simulink model "PROYECTO_IV_SIMULINK_II"  (R2020b)
settings: Solver=VariableStepAuto  StartTime=0.0  StopTime=500  RelTol=1e-3
libraries: simulink x1, pid_lib x1
settings Model: Creator=NITRO  LastModifiedBy=NITRO

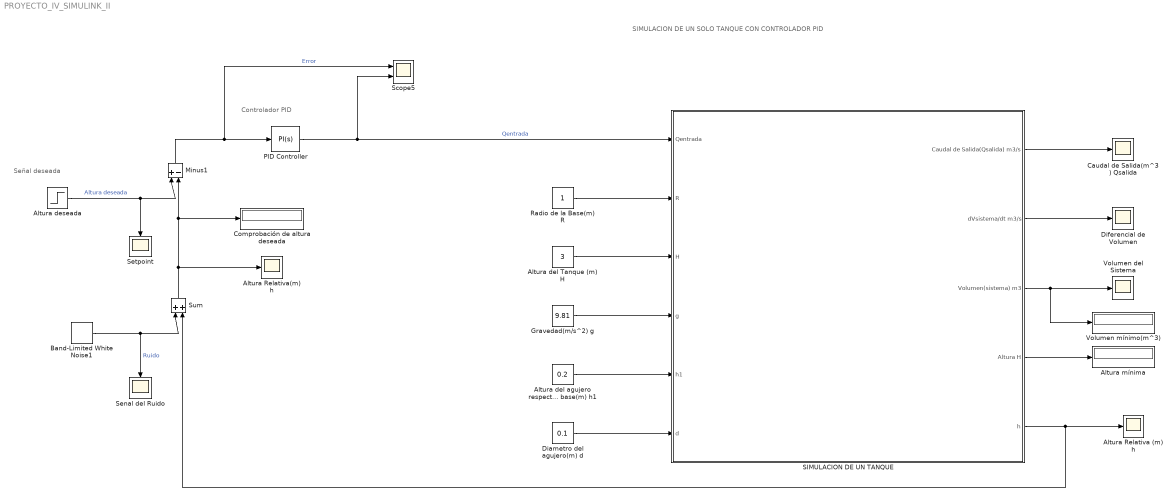
== system PROYECTO_IV_SIMULINK_II ==
  note: SIMULACION DE UN SOLO TANQUE CON CONTROLADOR PID
  note: Señal deseada
  note: Controlador PID
  Altura Relativa (m) h : Scope
  Altura Relativa(m) h : Scope
  Altura del Tanque (m) H : Constant  Value=3
  Altura del agujero respecto de la base(m) h1 : Constant  Value=0.2
  Altura deseada : Step  Time=50  Before=2  After=2.5  SampleTime=0
  Altura mínima : Display
  Band-Limited White Noise1 : simulink/Sources/Band-Limited White Noise  Cov=[0.001]  Ts=0.5  seed=[2525]
  Caudal de Salida(m^3) Qsalida : Scope
  Comprobación de altura deseada : Display
  Diametro del agujero(m) d : Constant  Value=0.1
  Diferencial de Volumen : Scope
  "Gravedad(m/s^2) g " : Constant  Value=9.81
  Minus1 : Sum  Inputs=|+-
  PID Controller : pid_lib/PID Controller  Controller=PI  Form=Parallel  TimeDomain=Continuous-time  UseExternalTs=off  SampleTime=-1  IntegratorMethod=Forward Euler  FilterMethod=Forward Euler  ControllerParametersSource=internal  P=10  I=4  D=0  UseFilter=on  N=0.0363987705373883  TunerSelectOption=Transfer Function Based (PID Tuner App)  InitialConditionSource=internal  InitialConditionForIntegrator=0  InitialConditionForFilter=0  DifferentiatorICPrevScaledInput=0  ExternalReset=none  TrackingMode=off  Kt=1  LimitOutput=on  SatLimitsSource=internal  UpperSaturationLimit=2000  LowerSaturationLimit=0  LinearizeAsGain=on  AntiWindupMode=none  Kb=1  POutMin=[]  POutMax=[]  IOutMin=[]  IOutMax=[]  DOutMin=[]  DOutMax=[]  NOutMin=[]  NOutMax=[]  SumOutMin=[]  SumOutMax=[]  SaturationOutMin=[]  SaturationOutMax=[]  PParamMin=[]  PParamMax=[]  IParamMin=[]  IParamMax=[]  DParamMin=[]  DParamMax=[]  NParamMin=[]  NParamMax=[]  KbParamMin=[]  KbParamMax=[]  KtParamMin=[]  KtParamMax=[]  KbOutMin=[]  KbOutMax=[]  KtOutMin=[]  KtOutMax=[]  IntegratorOutMin=[]  IntegratorOutMax=[]  FilterOutMin=[]  FilterOutMax=[]  SumI1OutMin=[]  SumI1OutMax=[]  SumI2OutMin=[]  SumI2OutMax=[]  SumI3OutMin=[]  SumI3OutMax=[]  SumI4OutMin=[]  SumI4OutMax=[]  SumDOutMin=[]  SumDOutMax=[]  DifferentiatorOutMin=[]  DifferentiatorOutMax=[]  FilterDiffOutCoefMin=[]  FilterDiffOutCoefMax=[]  ReciprocalOutMin=[]  ReciprocalOutMax=[]  SumDenOutMin=[]  SumDenOutMax=[]  SumNumOutMin=[]  SumNumOutMax=[]  DivideOutMin=[]  DivideOutMax=[]  UdiffTsProdOutMin=[]  UdiffTsProdOutMax=[]  NTsProdOutMin=[]  NTsProdOutMax=[]  UintegralTsProdOutMin=[]  UintegralTsProdOutMax=[]  UngainTsProdOutMin=[]  UngainTsProdOutMax=[]  IntegratorContinuousStateAttributes=''  IntegratorStateMustResolveToSignalObject=off  IntegratorRTWStateStorageClass=Auto  FilterContinuousStateAttributes=''  FilterStateMustResolveToSignalObject=off  FilterRTWStateStorageClass=Auto  ParallelPVariant=InternalParameters  IdealPVariant=Disabled  IVariant=InternalParameters  DVariant=Disabled  IntegratorVariant=Continuous  SatVariant=Enabled  AWVariant=Passthrough  PCopyVariant=Disabled  TRVariant=Disabled  FdbkBlocksVariant=Forward  IdealPFdbkVariant=Disabled  SatFdbkVariant=Disabled  DerivativeFilterVariant=Disabled  NVariant=Disabled  NCopyVariant=Disabled_SignalSpec  FilterICVariant=Disabled  IntegratorICVariant=InternalICs  ExternalResetVariant=Disabled  TRSumVariant=Passthrough  SumFdbkVariant=Disabled  SumVariant=Sum_PI  TsampFilterVariant=InternalTs  TsampNgainVariant=Passthrough  TsampIntegralVariant=Passthrough  ExternalSaturationOutDataTypeStr=Inherit: Same as second input
  Radio de la Base(m) R : Constant
  SIMULACION DE UN TANQUE : Subsystem
      mask Display: image('$imagefile'); % Use "Edit Image" on toolstrip to change.
  Scope5 : Scope  NumInputPorts=2
  Senal del Ruido : Scope
  Setpoint : Scope
  Sum : Sum  Inputs=|++
  Volumen del Sistema : Scope
  Volumen mínimo(m^3) : Display
  wires:
  SIMULACION DE UN TANQUE/3(Volumen(sistema) m3) -> Volumen mínimo(m^3)/1, Volumen del Sistema/1
  Radio de la Base(m) R/1 -> SIMULACION DE UN TANQUE/2(R)
  Altura del Tanque (m) H/1 -> SIMULACION DE UN TANQUE/3(H)
  "Gravedad(m/s^2) g "/1 -> SIMULACION DE UN TANQUE/4(g)
  Altura del agujero respecto de la base(m) h1/1 -> SIMULACION DE UN TANQUE/5(h1)
  Diametro del agujero(m) d/1 -> SIMULACION DE UN TANQUE/6(d)
  SIMULACION DE UN TANQUE/2(dVsistema/dt m3/s) -> Diferencial de Volumen/1
  SIMULACION DE UN TANQUE/1(Caudal de Salida(Qsalida) m3/s) -> Caudal de Salida(m^3) Qsalida/1
  SIMULACION DE UN TANQUE/5(h) -> Altura Relativa (m) h/1, Sum/2
  Minus1/1 -> Scope5/1, PID Controller/1  "Error"
  SIMULACION DE UN TANQUE/4(Altura H) -> Altura mínima/1
  Band-Limited White Noise1/1 -> Sum/1, Senal del Ruido/1  "Ruido"
  Altura deseada/1 -> Minus1/1, Setpoint/1  "Altura deseada"
  PID Controller/1 -> SIMULACION DE UN TANQUE/1(Qentrada), Scope5/2  "Qentrada"
  Sum/1 -> Minus1/2, Comprobación de altura deseada/1, Altura Relativa(m) h/1

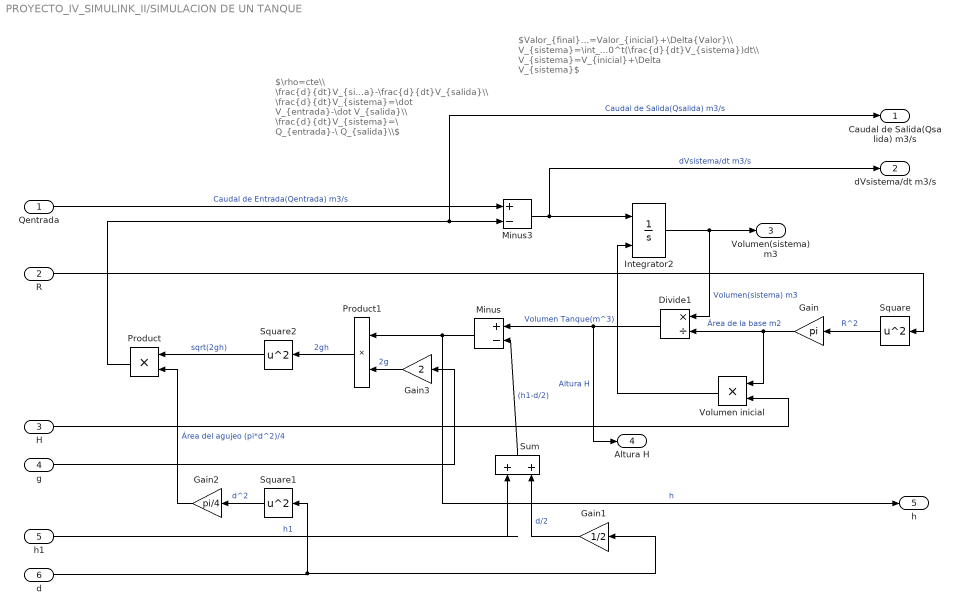
== system PROYECTO_IV_SIMULINK_II/SIMULACION DE UN TANQUE ==
  note: $\rho=cte\\ \frac{d}{dt}V_{sistema}=\frac{d}{dt}V_{entrada}-\frac{d}{dt}V_{salida}\\ \frac{d}{dt}V_{sistema}=\dot V_{entrada}-\dot V_{salida}\\ \frac{d}{dt}V_{sistema}=\ Q_{entrada}-\ Q_{salida}\\$
  note: $Valor_{final}=Valor_{inicial}+\Delta{Valor}\\ V_{sistema}=\int_0^t(\frac{d}{dt}V_{sistema})dt\\ V_{sistema}=V_{inicial}+\Delta V_{sistema}$
  Qentrada : Inport
  R : Inport  Port=2
  H : Inport  Port=3
  g : Inport  Port=4
  h1 : Inport  Port=5
  d : Inport  Port=6
  Divide1 : Product  Inputs=*/
  Gain : Gain  Gain=pi
  Gain1 : Gain  Gain=1/2
  Gain2 : Gain  Gain=pi/4
  Gain3 : Gain  Gain=2
  Integrator2 : Integrator  InitialConditionSource=external
  Minus : Sum  Inputs=+-
  Minus3 : Sum  Inputs=+-
  Product : Product
  Product1 : Product
  Square : Math  Operator=square  SaturateOnIntegerOverflow=on
  Square1 : Math  Operator=square  SaturateOnIntegerOverflow=on
  Square2 : Math  Operator=square  SaturateOnIntegerOverflow=on
  Sum : Sum  Inputs=|++
  Volumen inicial : Product
  Caudal de Salida(Qsalida) m3/s : Outport
  dVsistema/dt m3/s : Outport  Port=2
  Volumen(sistema) m3 : Outport  Port=3
  Altura H : Outport  Port=4
  h : Outport  Port=5
  wires:
  Square1/1 -> Gain2/1  "d^2"
  Divide1/1 -> Altura H/1, Minus/1  "Altura H"
  Square/1 -> Gain/1  "R^2"
  Minus/1 -> Product1/1, h/1  "h"
  d/1 -> Square1/1, Gain1/1
  Gain1/1 -> Sum/2  "d/2"
  Volumen inicial/1 -> Integrator2/2  "Volumen Tanque(m^3)"
  Integrator2/1 -> Volumen(sistema) m3/1, Divide1/1  "Volumen(sistema) m3"
  Gain3/1 -> Product1/2  "2g"
  Gain/1 -> Volumen inicial/1, Divide1/2  "Área de la base m2"
  Product1/1 -> Square2/1  "2gh"
  h1/1 -> Sum/1  "h1"
  Sum/1 -> Minus/2  "(h1-d/2)"
  g/1 -> Gain3/1
  Minus3/1 -> dVsistema/dt m3/s/1, Integrator2/1  "dVsistema/dt m3/s"
  Square2/1 -> Product/1  "sqrt(2gh)"
  R/1 -> Square/1
  Product/1 -> Caudal de Salida(Qsalida) m3/s/1, Minus3/2  "Caudal de Salida(Qsalida) m3/s"
  Gain2/1 -> Product/2  "Área del agujeo (pi*d^2)/4"
  Qentrada/1 -> Minus3/1  "Caudal de Entrada(Qentrada) m3/s"
  H/1 -> Volumen inicial/2
